simulink model "ConverterTestSim"  (R2024a)
settings: Solver=FixedStepAuto  StartTime=0.0  StopTime=50  FixedStep=0.0001  RelTol=1e-3
libraries: simulink x1
settings Model: Creator=Henrique Mesquita  LastModifiedBy=Henrique Mesquita

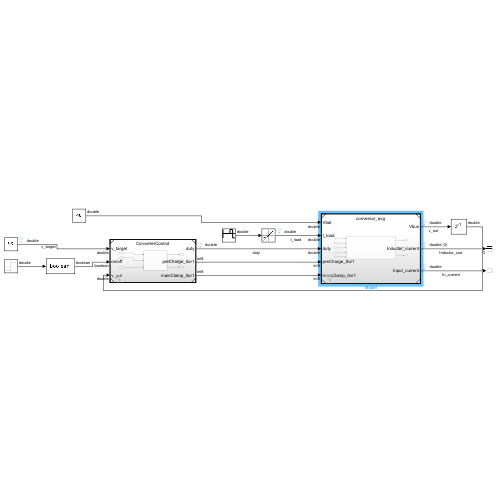
[thumbnail: Simulink's stored preview of the top-level diagram]
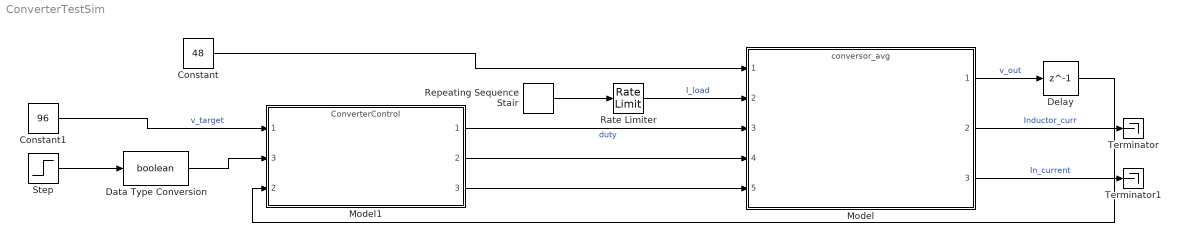
== system ConverterTestSim ==
  Constant : Constant  Value=48
  Constant1 : Constant  Value=96
  Data Type Conversion : DataTypeConversion  OutDataTypeStr=boolean  SaturateOnIntegerOverflow=off  RndMeth=Floor
  Delay : Delay  DelayLength=1
  Model : ModelReference  ModelNameDialog=conversor_avg.slx  SimulationMode=Normal  ModelReferenceVersion=4.8
  Model1 : ModelReference  ModelNameDialog=ConverterControl.slx  SimulationMode=Normal  ModelReferenceVersion=1.9
      settings: PortSchema="{\"entries\":[{\"content\":{\"sides\":[{\"content\":{\"connectorIds\":[\"In1\",\"In3\",\"In2\"]},\"type\":\"ConnectorPlacement.EquallySpacedRectSide\",\"uuid\":\"68b399cf-a5dd-481e-9a31-f4bea2a0363b\"},{\"content\":{\"connectorIds\":[\"Out1\",\"Out2\",\"Out3\"],\"side\":\"RIGHT\"},\"type\":\"ConnectorPlacement.EquallySpacedRectSide\",\"uuid\":\"1da21c56-f709-47ef-b5ca-3a66b7214b38\"},{\"content\":{\"side\":\"TOP\"},\"type\":\"ConnectorPlacement.EquallySpacedRectSide\",\"uuid\":\"8c99eeb7-d6aa-4e4c-9eef-bda626ec3e36\"}]},\"type\":\"ConnectorPlacement.EquallySpacedConnector\",\"uuid\":\"d58d2baf-62b7-4f99-ae7d-cb296a23b1bb\"}],\"packageUris\":[\"http://schema.mathworks.com/mf0/Connector/R2020b\"],\"version\":\"1.0\"}"
  Rate Limiter : RateLimiter  RisingSlewLimit=5000  FallingSlewLimit=-5000
  Repeating Sequence Stair : simulink/Sources/Repeating Sequence Stair  OutValues=[0 0.1 10 200 -200].'  tsamp=10  OutMin=[]  OutMax=[]  OutDataTypeStr=double  OutputDataTypeScalingMode=double  OutDataType=fixdt(0,8)  ConRadixGroup=Best Precision: Vector-wise  OutScaling=2^-12
  Step : Step  Time=0.5  SampleTime=0
  Terminator : Terminator
  Terminator1 : Terminator
  wires:
  Model1/1 -> Model/3  "duty"
  Model/1 -> Delay/1  "v_out"
  Model/2 -> Terminator/1  "Inductor_curr"
  Constant/1 -> Model/1
  Repeating Sequence Stair/1 -> Rate Limiter/1
  Rate Limiter/1 -> Model/2  "I_load"
  Constant1/1 -> Model1/1  "v_target"
  Model/3 -> Terminator1/1  "In_current"
  Step/1 -> Data Type Conversion/1
  Model1/2 -> Model/4
  Model1/3 -> Model/5
  Data Type Conversion/1 -> Model1/3
  Delay/1 -> Model1/2
